simulink model "PANCLctx"  (R2020a)
settings: Solver=ode3  StartTime=0.0  StopTime=10.0  FixedStep=0.1  RelTol=1e-3  EnableMultiTasking=on
settings Model: Creator=adeca  LastModifiedBy=Arnaldo
settings DataIOCC: LimitDataPoints=on  SaveFormat=Array  SignalLoggingSaveFormat=ModelDataLogs  ReturnWorkspaceOutputs=off
settings OptimizationCC: ExpressionDepthLimit=2147483647  InitFltsAndDblsToZero=on  LifeSpan=inf
settings DebuggingCC: UnderspecifiedInitializationDetection=Classic  MergeDetectMultiDrivingBlocksExec=none  SolverPrmCheckMsg=warning  FcnCallInpInsideContextMsg=warning  StateNameClashWarn=warning  SFUnexpectedBacktrackingDiag=warning  SFNoUnconditionalDefaultTransitionDiag=warning  SFExecutionAtInitializationDiag=none  ArithmeticOperatorsInVariantConditions=warning
settings HardwareCC: ProdBitPerPointer=32  ProdBitPerSizeT=32  ProdBitPerPtrDiffT=32  ProdLargestAtomicFloat=None  ProdIntDivRoundTo=Undefined  ProdEndianess=Unspecified  ProdWordSize=32  ProdHWDeviceType=32-bit Generic
settings ModelReferenceCC: PropagateSignalLabelsOutOfModel=off
settings SFSimCC: SimUseLocalCustomCode=off  CustomCodeUndefinedFunction=UseInterfaceOnly
settings RTWCC: RTWUseLocalCustomCode=off
settings CodeAppCC: StateflowObjectComments=on
settings GRTTargetCC: TargetLangStandard=C89/C90 (ANSI)  CombineOutputUpdateFcns=off  GRTInterface=on
settings ConfigComp: CovMetricSettings=dw  CovHtmlReporting=on  CovSaveCumulativeToWorkspaceVar=on  CovSaveSingleToWorkspaceVar=on  CovExternalEMLEnable=off

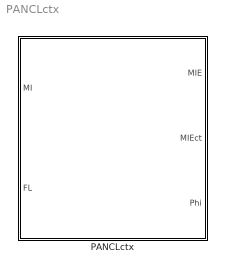
== system PANCLctx ==
  PANCLctx : Subsystem  Tag=NAP  Description=Célula de Aprendizagem NAP

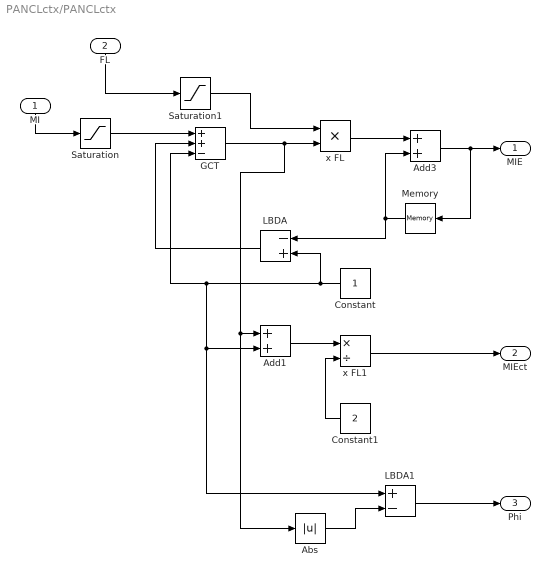
== system PANCLctx/PANCLctx ==
  MI : Inport
  FL : Inport  Port=2
  Abs : Abs
  Add1 : Sum
  Add3 : Sum
  Constant : Constant
  Constant1 : Constant  Value=2
  GCT : Sum  Inputs=++-
  LBDA : Sum  Inputs=-+
  LBDA1 : Sum  Inputs=+-
  Memory : Memory  InitialCondition=0.5  LinearizeAsDelay=on
  Saturation : Saturate  UpperLimit=1  LowerLimit=0
  Saturation1 : Saturate  UpperLimit=1  LowerLimit=0
  x FL : Product  Inputs=**
  x FL1 : Product  Inputs=*/
  MIE : Outport
  MIEct : Outport  Port=2
  Phi : Outport  Port=3
  wires:
  MI/1 -> Saturation/1
  x FL/1 -> Add3/1
  Memory/1 -> Add3/2, LBDA/1
  Add3/1 -> Memory/1, MIE/1
  LBDA/1 -> GCT/2
  Constant/1 -> LBDA/2, Add1/2, LBDA1/1, GCT/3
  GCT/1 -> Abs/1, Add1/1, x FL/2
  FL/1 -> Saturation1/1
  Add1/1 -> x FL1/1
  Constant1/1 -> x FL1/2
  x FL1/1 -> MIEct/1
  Abs/1 -> LBDA1/2
  LBDA1/1 -> Phi/1
  Saturation/1 -> GCT/1
  Saturation1/1 -> x FL/1
